simulink model "efterKirsten"  (R2015a)
settings: Solver=ode3  StartTime=0.0  StopTime=20  FixedStep=.01  RelTol=1e-3
libraries: cstblocks x7, simulink x3
settings Model: Creator=morten  LastModifiedBy=morten

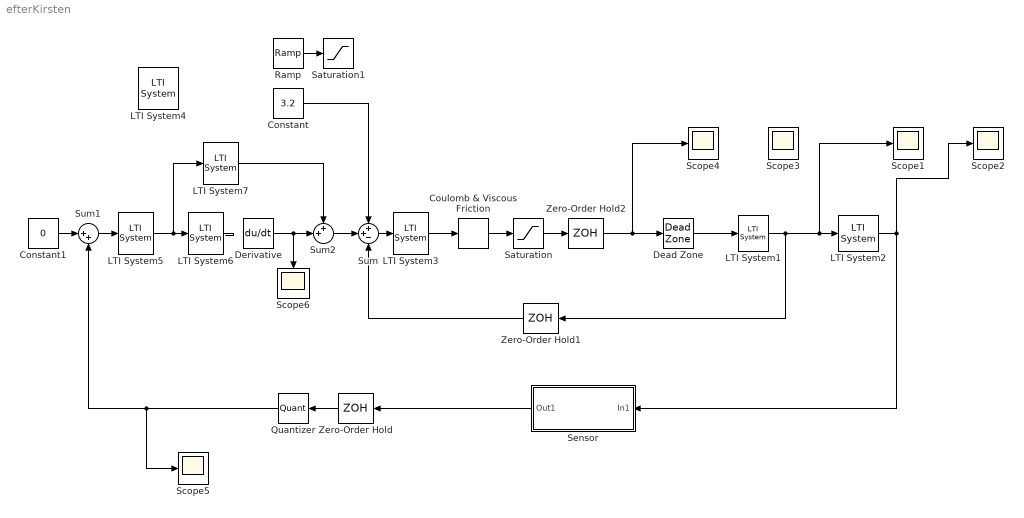
== system efterKirsten ==
  Constant : Constant  Value=3.2
  Constant1 : Constant  Value=0
  Coulomb & Viscous Friction : simulink/Discontinuities/Coulomb & Viscous Friction  offset=4.5  gain=1
  Dead Zone : DeadZone  LowerValue=-4.5  UpperValue=4.5  SaturateOnIntegerOverflow=on
  Derivative : Derivative
  LTI System1 : cstblocks/LTI System  sys=Xm  IC=[]
  LTI System2 : cstblocks/LTI System  sys=Wm  IC=[]
  LTI System3 : cstblocks/LTI System  sys=C1  IC=[]
  LTI System4 : cstblocks/LTI System  sys=dC2  IC=[]
  LTI System5 : cstblocks/LTI System  sys=k  IC=[]
  LTI System6 : cstblocks/LTI System  sys=td  IC=[]
  LTI System7 : cstblocks/LTI System  sys=tp  IC=[]
  Quantizer : Quantizer  QuantizationInterval=0.001  LinearizeAsGain=off
  Ramp : simulink/Sources/Ramp  slope=.5  start=0  X0=0
  Saturation : Saturate  UpperLimit=12.5  LowerLimit=-12.5
  Saturation1 : Saturate  UpperLimit=3.2  LowerLimit=0
  Scope{1..6} (6 alike) : Scope
      Scope2 settings: TimeRange=40  YMin=-0.085  YMax=0.015  SaveName=ScopeData2
      Scope4 settings: SaveName=ScopeData3
      Scope5 settings: YMin=-0.085  YMax=0.015  SaveName=ScopeData4
      Scope6 settings: YMin=-0.085  YMax=0.015  SaveName=ScopeData5
  Sensor : Subsystem
  Sum : Sum  Inputs=++-
  Sum1 : Sum  Inputs=|++
  Sum2 : Sum  Inputs=++|
  Zero-Order Hold : ZeroOrderHold  SampleTime=.01
  Zero-Order Hold1 : ZeroOrderHold  SampleTime=.01
  Zero-Order Hold2 : ZeroOrderHold  SampleTime=.01
  wires:
  LTI System1/1 -> LTI System2/1, Scope1/1, Zero-Order Hold1/1
  Constant1/1 -> Sum1/1
  Coulomb & Viscous Friction/1 -> Saturation/1
  LTI System2/1 -> Sensor/1(In1), Scope2/1
  Sensor/1(Out1) -> Zero-Order Hold/1
  Constant/1 -> Sum/1
  Ramp/1 -> Saturation1/1
  Sum1/1 -> LTI System5/1
  Quantizer/1 -> Scope5/1, Sum1/2
  Sum/1 -> LTI System3/1
  LTI System3/1 -> Coulomb & Viscous Friction/1
  Saturation/1 -> Zero-Order Hold2/1
  Dead Zone/1 -> LTI System1/1
  Derivative/1 -> Sum2/2, Scope6/1
  LTI System5/1 -> LTI System7/1, LTI System6/1
  LTI System6/1 -> ?
  Sum2/1 -> Sum/2
  LTI System7/1 -> Sum2/1
  Zero-Order Hold/1 -> Quantizer/1
  Zero-Order Hold1/1 -> Sum/3
  Zero-Order Hold2/1 -> Dead Zone/1, Scope4/1

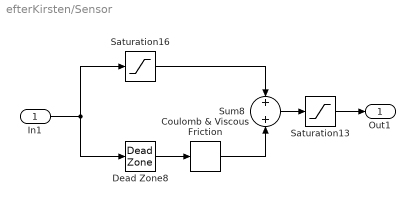
== system efterKirsten/Sensor ==
  In1 : Inport
  Coulomb & Viscous Friction : simulink/Discontinuities/Coulomb & Viscous Friction  offset=[0.165]  gain=1
  Dead Zone8 : DeadZone  LowerValue=-0.3225  UpperValue=0.337  SaturateOnIntegerOverflow=on
  Saturation13 : Saturate  UpperLimit=0.664  LowerLimit=-0.68
  Saturation16 : Saturate  UpperLimit=.1627  LowerLimit=-0.1787
  Sum8 : Sum  Inputs=+|+
  Out1 : Outport
  wires:
  In1/1 -> Saturation16/1, Dead Zone8/1
  Dead Zone8/1 -> Coulomb & Viscous Friction/1
  Sum8/1 -> Saturation13/1
  Saturation16/1 -> Sum8/1
  Coulomb & Viscous Friction/1 -> Sum8/2
  Saturation13/1 -> Out1/1
